simulink model "pv_wind_hybrid"  (R2024a)
settings: Solver=VariableStepAuto  StartTime=0.0  StopTime=1  RelTol=1e-3
libraries: spsSeriesRLCBranchLib x24, spsIGBTDiodeLib x12, spsDiodeLib x7, spsSawtoothGeneratorLib x6, spsGroundLib x5, spsThreePhaseVIMeasurementLib x5, spsCurrentMeasurementLib x4, spsVoltageMeasurementLib x3, spspowerguiLib x2, spsIGBTLib x1, spsPVArrayLib x1, eePwmGenerator x1
settings Model: Creator=91889  LastModifiedBy=91889
settings SolverCC: ZeroCrossAlgorithm=Adaptive

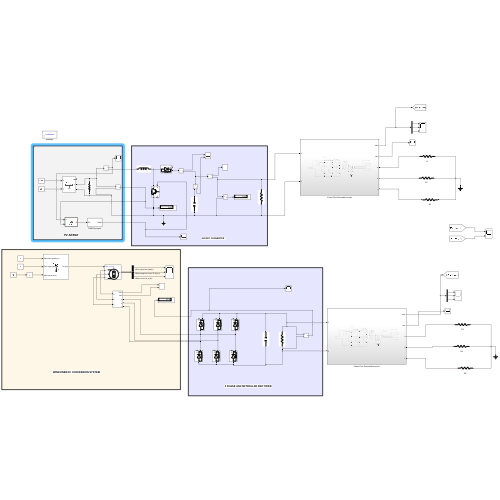
[thumbnail: Simulink's stored preview of the top-level diagram]
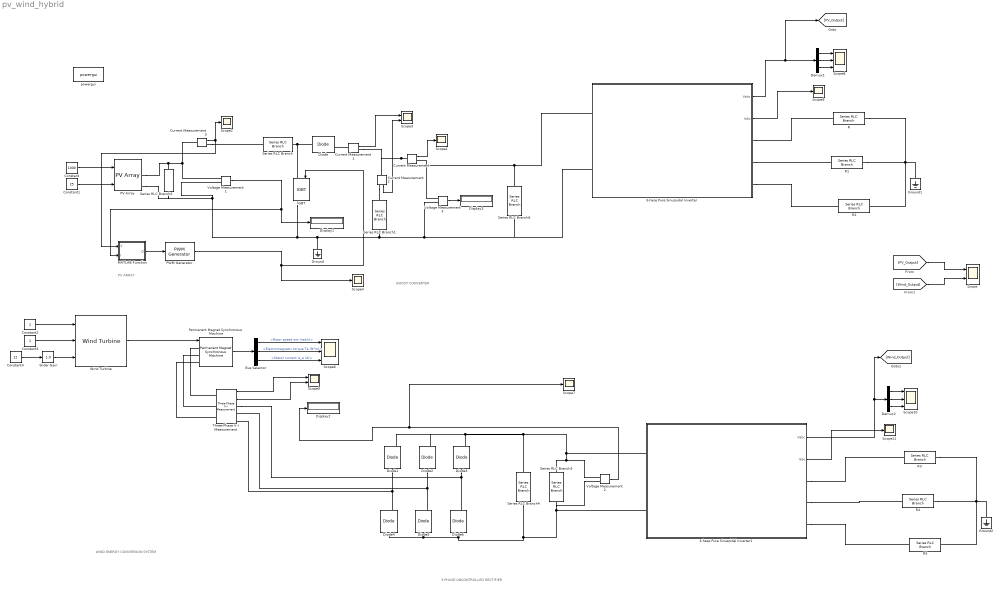
== system pv_wind_hybrid ==
  note: 3 PHASE UNCONTROLLED RECTIFIER
  note: WIND ENERGY CONVERSION SYSTEM
  note: BOOST CONVERTER
  note: PV ARRAY
  3-hase Pure Sinusoidal Inverter : Subsystem
  3-hase Pure Sinusoidal Inverter1 : Subsystem
  Bus Selector : BusSelector  OutputSignals=Rotor speed wm (rad/s),Electromagnetic torque Te (N*m),Stator current is_a (A)
  Constant : Constant  Value=1000
  Constant1 : Constant  Value=25
  Constant2 : Constant
  Constant3 : Constant
  Constant4 : Constant  Value=12
  Current Measurement{,1..3} (4 alike) : spsCurrentMeasurementLib/Current Measurement  PhasorSimulation=off  OutputType=Complex  PSBequivalent=0
  Demux1 : Demux  Outputs=3
  Demux2 : Demux  Outputs=3
  Diode{,1..6} (7 alike) : spsDiodeLib/Diode  Ron=0.001  Lon=0  Vf=0.8  IC=0  UseSnubber=0  Rs=500  Cs=250e-9  Measurements=on
  Display1 : Display
  Display2 : Display
  Display3 : Display
  Ground : spsGroundLib/Ground  LConnTagsString=a
  Ground1 : spsGroundLib/Ground  LConnTagsString=a
  Ground2 : spsGroundLib/Ground  LConnTagsString=a
  IGBT : spsIGBTLib/IGBT  Ron=0.001  Lon=0  Vf=1  Tf=1e-6  Tt=2e-6  IC=0  Rs=1e5  Cs=inf  Measurements=on
  MATLAB Function : MATLAB Function  TreatAsAtomicUnit=on
  PV Array : spsPVArrayLib/PV Array  Npar=1  Nser=1  PlotType=array @ 1000 W/m2 & specified temperatures  S_vec="[ 1000  500  100 ]"  Temp_C_vec="[ 45 25  ]"  ModuleName=User-defined  PlotWhenSelected=off  Pm=39.648  Ncell=36  Voc=21.6  Isc=2.55  Vm=16.8  Im=2.36  beta_Voc_pc=-0.36099  alpha_Isc_pc=0.102  beta_Voc=-0.077974  alpha_Isc=0.002601  IL=2.5568  I0=9.4856e-11  nI=0.97333  Rsh=355.4065  Rs=0.94376  RobustModel=off  RobustCellTemperature=313.3991  BAL=on  Tc=1e-6  Tfilter=5e-5
      link override Diode Rsh/Transfer Fcn: Numerator=10  Denominator=5e-1
  PWM Generator : eePwmGenerator/PWM Generator  CarrCount=Up  Tper=0.001  Tdelay=0  Ts=5e-5
  Permanent Magnet Synchronous Machine : spsPermanentMagnetSynchronousMachineLib/Permanent Magnet Synchronous Machine  NbPhases=3  FluxDistribution=Sinusoidal  RotorType=Round  MechanicalLoad=Torque Tm  PresetModel=No  ShowDetailedParameters=on  MeasurementBus=off  Resistance=0.0485  Inductance=8.5e-3  dqInductances=[8.5e-3,8.5e-3]  La=0.000395  MachineConstant=Flux linkage established by magnets (V.s)  Flux=0.1194  VoltageCst=86.6271  TorqueCst=0.7164  Flat=120  Mechanical=[0.0027 0.0004924 4 0]  PolePairs=4  InitialConditions=[0,0, 0,0]  InitialConditions5ph=[0 0 0 0 0 0]  RefAngle=90 degrees behind phase A axis (modified Park)  IterativeDiscreteModel=Trapezoidal non iterative  TsBlock=-1  TsPowergui=0
  R{,1..5} (6 alike) : spsSeriesRLCBranchLib/Series RLC Branch  LConnTagsString=__new0  RConnTagsString=__new0  BranchType=R  Resistance=10  Inductance=1e-3  SetiL0=off  InitialCurrent=0  Capacitance=1e-6  Setx0=off  InitialVoltage=0  Measurements=None
  Scope : Scope  NumInputPorts=2
  Scope{1..2,4,7,9,11} (6 alike) : Scope
  Scope10 : Scope  NumInputPorts=3
  Scope3 : Scope  NumInputPorts=2
  Scope5 : Scope  NumInputPorts=2
  Scope6 : Scope  NumInputPorts=3
  Scope8 : Scope  NumInputPorts=3
  Series RLC Branch : spsSeriesRLCBranchLib/Series RLC Branch  LConnTagsString=__new0  RConnTagsString=__new0  BranchType=L  Resistance=1  Inductance=32e-3  SetiL0=off  InitialCurrent=0  Capacitance=1e-6  Setx0=off  InitialVoltage=0  Measurements=None
  Series RLC Branch1 : spsSeriesRLCBranchLib/Series RLC Branch  LConnTagsString=__new0  RConnTagsString=__new0  BranchType=C  Resistance=1  Inductance=1e-3  SetiL0=off  InitialCurrent=0  Capacitance=1000e-6  Setx0=off  InitialVoltage=0  Measurements=None
  Series RLC Branch2 : spsSeriesRLCBranchLib/Series RLC Branch  LConnTagsString=__new0  RConnTagsString=__new0  BranchType=R  Resistance=200  Inductance=1e-3  SetiL0=off  InitialCurrent=0  Capacitance=1e-6  Setx0=off  InitialVoltage=0  Measurements=None
  Series RLC Branch3 : spsSeriesRLCBranchLib/Series RLC Branch  LConnTagsString=__new0  RConnTagsString=__new0  BranchType=R  Resistance=100  Inductance=1e-3  SetiL0=off  InitialCurrent=0  Capacitance=1e-6  Setx0=off  InitialVoltage=0  Measurements=None
  Series RLC Branch4 : spsSeriesRLCBranchLib/Series RLC Branch  LConnTagsString=__new0  RConnTagsString=__new0  BranchType=C  Resistance=1  Inductance=1e-3  SetiL0=off  InitialCurrent=0  Capacitance=1e-6  Setx0=off  InitialVoltage=0  Measurements=None
  Series RLC Branch6 : spsSeriesRLCBranchLib/Series RLC Branch  LConnTagsString=__new0  RConnTagsString=__new0  BranchType=R  Resistance=10  Inductance=1e-3  SetiL0=off  InitialCurrent=0  Capacitance=32e-6  Setx0=off  InitialVoltage=0  Measurements=None
  Slider Gain : simulink/Math Operations/Slider Gain  gain=1.0  low=0.5  high=1
  Three-Phase V-I Measurement : spsThreePhaseVIMeasurementLib/Three-Phase V-I Measurement  VoltageMeasurement=phase-to-phase  SetLabelV=off  LabelV=Vabc  Vpu=off  VpuLL=off  CurrentMeasurement=yes  SetLabelI=off  LabelI=Iabc  Ipu=off  Pbase=100e6  Vbase=500e3  OutputType=Complex  PhasorSimulation=off  PSBequivalent=0
  Voltage Measurement1 : spsVoltageMeasurementLib/Voltage Measurement  PhasorSimulation=off  OutputType=Complex  PSBequivalent=0
  Voltage Measurement2 : spsVoltageMeasurementLib/Voltage Measurement  PhasorSimulation=off  OutputType=Complex  PSBequivalent=0
  Voltage Measurement3 : spsVoltageMeasurementLib/Voltage Measurement  PhasorSimulation=off  OutputType=Complex  PSBequivalent=0
  Wind Turbine : spsWindTurbineLib/Wind Turbine  Pnom=1.5e6  Pelec_base=1.5e6/0.9  wind_base=12  P_wind_base=0.73  speed_nom=1.2  pitch_angle=0  c1_c6="[0.51763          116          0.4            5           21     0.006795]"  cp_nom=0.48  lambda_nom=8.1
  powergui : sps_lib/powergui  Priority=1  SimulationMode=Continuous  SampleTime=50e-6  frequency=60  Iterations=50  frequencyindice=0  Pbase=100e6  ErrMax=1e-4  UnitsV=kV  UnitsW=MW  buscounter=0  FunctionMessages=off  echomessages=off  EnableUseOfTLC=off  CurrentSourceSwitches=off  DisableSnubberDevices=off  DisableRonSwitches=off  DisableVfSwitches=off  DisplayEquations=off  AutomaticDiscreteSolvers=off  SolverType=Tustin/Backward Euler (TBE)  Interpol=off  ExternalGateDelay=off  methode=off  Ts=100  x0status=blocks  SPID=on  SwTol=0  HookPort=off  NonlinearTolerance=1e-4  nMaxIteration=100  ContinueOnMaxIteration=off  RestoreLinks=warning  ResistiveCurrentMeasurement=off  Frange=[0:2:500]  Ylog=off  Xlog=on  ShowGrid=off  save=off  variable=ZData  structure=0  ZoomFFT=off  StartTime=0.0  cycles=1  DisplayStyle=1  fundamental=60  FreqAxis=off  MaxFrequency=1000  frequencyindicesteady=1  RmsSteady=1  display=off
  wires:
  Current Measurement1/1 -> Scope3/1
  Current Measurement2/1 -> Scope3/2
  Current Measurement/1 -> Scope1/1
  Current Measurement3/1 -> Scope2/1, MATLAB Function/1(V)
  Constant/1 -> PV Array/1
  Constant1/1 -> PV Array/2
  Voltage Measurement1/1 -> MATLAB Function/2(I), Display1/1
  MATLAB Function/1(D) -> PWM Generator/1
  PWM Generator/1 -> Scope4/1, IGBT/1
  Bus Selector/2 -> Scope6/2  "<Electromagnetic torque Te (N*m)>"
  Bus Selector/3 -> Scope6/3  "<Stator current is_a (A)>"
  Constant4/1 -> Slider Gain/1
  Wind Turbine/1 -> Permanent Magnet Synchronous Machine/1
  Three-Phase V-I Measurement/2 -> Scope5/2
  Constant3/1 -> Wind Turbine/2
  Three-Phase V-I Measurement/1 -> Scope5/1
  Slider Gain/1 -> Wind Turbine/3
  Bus Selector/1 -> Scope6/1  "<Rotor speed wm (rad/s)>"
  Permanent Magnet Synchronous Machine/1 -> Bus Selector/1
  Constant2/1 -> Wind Turbine/1
  Voltage Measurement2/1 -> Display2/1, Scope7/1
  3-hase Pure Sinusoidal Inverter/2(Iabc) -> Scope9/1
  Demux1/3 -> Scope8/3
  Demux1/1 -> Scope8/1
  3-hase Pure Sinusoidal Inverter/1(Vabc) -> [PV_Output], Demux1/1
  Demux1/2 -> Scope8/2
  3-hase Pure Sinusoidal Inverter1/1(Vabc) -> [Wind_Output], Demux2/1
  Demux2/2 -> Scope10/2
  Demux2/3 -> Scope10/3
  Demux2/1 -> Scope10/1
  3-hase Pure Sinusoidal Inverter1/2(Iabc) -> Scope11/1
  Voltage Measurement3/1 -> Display3/1
  [PV_Output] -> Scope/1
  [Wind_Output] -> Scope/2
  connections:
  Series RLC Branch/RConn1 -- IGBT/LConn1 -- Diode/LConn1
  Current Measurement/LConn1 -- Current Measurement2/LConn1 -- Current Measurement1/RConn1
  Current Measurement3/RConn1 -- Series RLC Branch/LConn1
  Current Measurement1/LConn1 -- Diode/RConn1
  PV Array/RConn1 -- Series RLC Branch2/LConn1 -- Voltage Measurement1/LConn1 -- Current Measurement3/LConn1
  Current Measurement2/RConn1 -- Series RLC Branch1/LConn1
  Three-Phase V-I Measurement/LConn1 -- Permanent Magnet Synchronous Machine/LConn1
  Three-Phase V-I Measurement/LConn3 -- Permanent Magnet Synchronous Machine/LConn3
  Three-Phase V-I Measurement/LConn2 -- Permanent Magnet Synchronous Machine/LConn2
  Diode1/LConn1 -- Diode4/RConn1 -- Three-Phase V-I Measurement/RConn3
  Diode2/LConn1 -- Three-Phase V-I Measurement/RConn2 -- Diode5/RConn1
  Diode3/LConn1 -- Three-Phase V-I Measurement/RConn1 -- Diode6/RConn1
  Series RLC Branch3/LConn1 -- 3-hase Pure Sinusoidal Inverter1/LConn1 -- Series RLC Branch4/LConn1 -- Diode1/RConn1 -- Diode2/RConn1 -- Diode3/RConn1 -- Voltage Measurement2/LConn1
  IGBT/RConn1 -- Series RLC Branch2/RConn1 -- PV Array/RConn2 -- Voltage Measurement1/LConn2 -- Ground/LConn1 -- Series RLC Branch6/RConn1 -- 3-hase Pure Sinusoidal Inverter/LConn2 -- Voltage Measurement3/LConn2 -- Series RLC Branch1/RConn1
  R1/RConn1 -- R2/RConn1 -- Ground1/LConn1 -- R/RConn1
  3-hase Pure Sinusoidal Inverter/RConn1 -- R/LConn1
  3-hase Pure Sinusoidal Inverter/RConn2 -- R1/LConn1
  3-hase Pure Sinusoidal Inverter/RConn3 -- R2/LConn1
  R4/RConn1 -- R5/RConn1 -- Ground2/LConn1 -- R3/RConn1
  3-hase Pure Sinusoidal Inverter1/RConn3 -- R5/LConn1
  3-hase Pure Sinusoidal Inverter1/RConn2 -- R4/LConn1
  3-hase Pure Sinusoidal Inverter1/RConn1 -- R3/LConn1
  3-hase Pure Sinusoidal Inverter/LConn1 -- Series RLC Branch6/LConn1 -- Voltage Measurement3/LConn1 -- Current Measurement/RConn1
  3-hase Pure Sinusoidal Inverter1/LConn2 -- Series RLC Branch4/RConn1 -- Diode4/LConn1 -- Diode5/LConn1 -- Diode6/LConn1 -- Series RLC Branch3/RConn1 -- Voltage Measurement2/LConn2

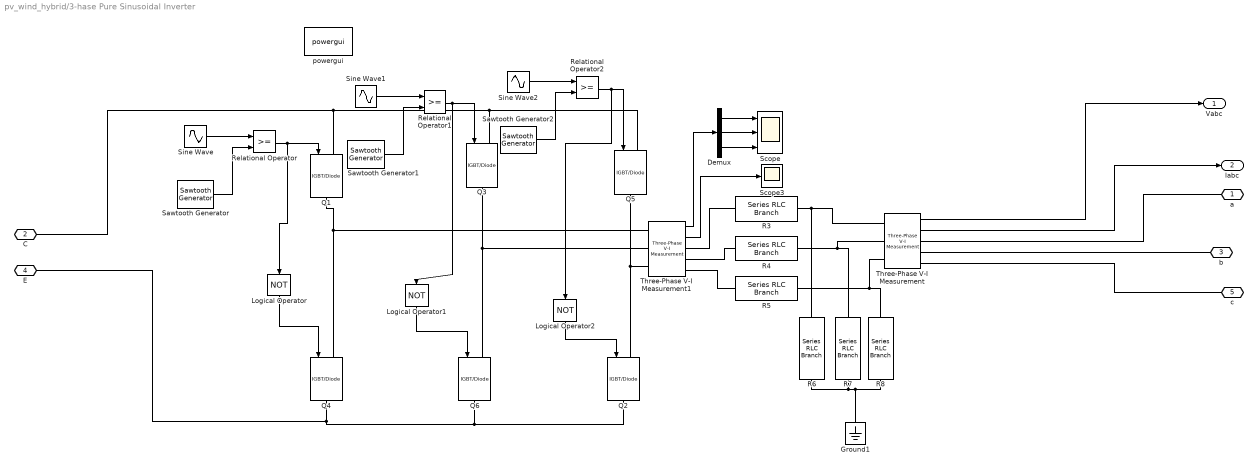
== system pv_wind_hybrid/3-hase Pure Sinusoidal Inverter ==
  Demux : Demux  Outputs=3
  Ground1 : spsGroundLib/Ground  LConnTagsString=a
  Logical Operator : Logic  Operator=NOT  AllPortsSameDT=off  OutDataTypeStr=boolean
  Logical Operator1 : Logic  Operator=NOT  AllPortsSameDT=off  OutDataTypeStr=boolean
  Logical Operator2 : Logic  Operator=NOT  AllPortsSameDT=off  OutDataTypeStr=boolean
  Q{1..6} (6 alike) : spsIGBTDiodeLib/IGBT//Diode  Ron=1e-3  Rs=1e5  Cs=inf  Measurements=off
  R3 : spsSeriesRLCBranchLib/Series RLC Branch  LConnTagsString=__new0  RConnTagsString=__new0  BranchType=L  Resistance=10  Inductance=80e-3  SetiL0=off  InitialCurrent=0  Capacitance=1e-6  Setx0=off  InitialVoltage=0  Measurements=None
  R4 : spsSeriesRLCBranchLib/Series RLC Branch  LConnTagsString=__new0  RConnTagsString=__new0  BranchType=L  Resistance=10  Inductance=80e-3  SetiL0=off  InitialCurrent=0  Capacitance=1e-6  Setx0=off  InitialVoltage=0  Measurements=None
  R5 : spsSeriesRLCBranchLib/Series RLC Branch  LConnTagsString=__new0  RConnTagsString=__new0  BranchType=L  Resistance=10  Inductance=80e-3  SetiL0=off  InitialCurrent=0  Capacitance=1e-6  Setx0=off  InitialVoltage=0  Measurements=None
  R6 : spsSeriesRLCBranchLib/Series RLC Branch  LConnTagsString=__new0  RConnTagsString=__new0  BranchType=C  Resistance=10  Inductance=80e-3  SetiL0=off  InitialCurrent=0  Capacitance=300e-6  Setx0=off  InitialVoltage=0  Measurements=None
  R7 : spsSeriesRLCBranchLib/Series RLC Branch  LConnTagsString=__new0  RConnTagsString=__new0  BranchType=C  Resistance=10  Inductance=80e-3  SetiL0=off  InitialCurrent=0  Capacitance=300e-6  Setx0=off  InitialVoltage=0  Measurements=None
  R8 : spsSeriesRLCBranchLib/Series RLC Branch  LConnTagsString=__new0  RConnTagsString=__new0  BranchType=C  Resistance=10  Inductance=80e-3  SetiL0=off  InitialCurrent=0  Capacitance=300e-6  Setx0=off  InitialVoltage=0  Measurements=None
  Relational Operator : RelationalOperator  OutDataTypeStr=boolean  InputSameDT=off
  Relational Operator1 : RelationalOperator  OutDataTypeStr=boolean  InputSameDT=off
  Relational Operator2 : RelationalOperator  OutDataTypeStr=boolean  InputSameDT=off
  Sawtooth Generator : spsSawtoothGeneratorLib/Sawtooth Generator  Freq=1000  Phase=180  Ts=0
  Sawtooth Generator1 : spsSawtoothGeneratorLib/Sawtooth Generator  Freq=1000  Phase=180  Ts=0
  Sawtooth Generator2 : spsSawtoothGeneratorLib/Sawtooth Generator  Freq=1000  Phase=180  Ts=0
  Scope : Scope  NumInputPorts=3
  Scope3 : Scope
  Sine Wave : Sin  Amplitude=0.9  Frequency=2*pi*50  SampleTime=0
  Sine Wave1 : Sin  Amplitude=0.9  Frequency=2*pi*50  Phase=120*(pi/180)  SampleTime=0
  Sine Wave2 : Sin  Amplitude=0.9  Frequency=2*pi*50  Phase=240*(pi/180)  SampleTime=0
  Three-Phase V-I Measurement : spsThreePhaseVIMeasurementLib/Three-Phase V-I Measurement  VoltageMeasurement=phase-to-phase  SetLabelV=off  LabelV=Vabc  Vpu=off  VpuLL=off  CurrentMeasurement=yes  SetLabelI=off  LabelI=Iabc  Ipu=off  Pbase=100e6  Vbase=500e3  OutputType=Complex  PhasorSimulation=off  PSBequivalent=0
  Three-Phase V-I Measurement1 : spsThreePhaseVIMeasurementLib/Three-Phase V-I Measurement  VoltageMeasurement=phase-to-phase  SetLabelV=off  LabelV=Vabc  Vpu=off  VpuLL=off  CurrentMeasurement=yes  SetLabelI=off  LabelI=Iabc  Ipu=off  Pbase=100e6  Vbase=500e3  OutputType=Complex  PhasorSimulation=off  PSBequivalent=0
  powergui : spspowerguiLib/powergui  Priority=1  SimulationMode=Continuous  SampleTime=50e-6  frequency=60  Iterations=50  frequencyindice=0  Pbase=100e6  ErrMax=1e-4  UnitsV=kV  UnitsW=MW  buscounter=0  FunctionMessages=off  echomessages=off  EnableUseOfTLC=off  CurrentSourceSwitches=off  DisableSnubberDevices=off  DisableRonSwitches=off  DisableVfSwitches=off  DisplayEquations=off  AutomaticDiscreteSolvers=off  SolverType=Tustin/Backward Euler (TBE)  Interpol=off  ExternalGateDelay=off  methode=off  Ts=100  x0status=blocks  SPID=off  SwTol=0  HookPort=off  NonlinearTolerance=1e-4  nMaxIteration=100  ContinueOnMaxIteration=off  RestoreLinks=warning  ResistiveCurrentMeasurement=off  Frange=[0:2:500]  Ylog=off  Xlog=on  ShowGrid=off  save=off  variable=ZData  structure=Vo  ZoomFFT=off  StartTime=0.0  cycles=1  DisplayStyle=1  fundamental=50  FreqAxis=on  MaxFrequency=1000  frequencyindicesteady=1  RmsSteady=1  display=off
  a : PMIOPort  Side=Right
  C : PMIOPort  Port=2  Side=Left
  b : PMIOPort  Port=3  Side=Right
  E : PMIOPort  Port=4  Side=Left
  c : PMIOPort  Port=5  Side=Right
  Vabc : Outport
  Iabc : Outport  Port=2
  wires:
  Relational Operator1/1 -> Q3/1, Logical Operator1/1
  Logical Operator/1 -> Q4/1
  Three-Phase V-I Measurement/1 -> Vabc/1
  Three-Phase V-I Measurement1/2 -> Scope3/1
  Logical Operator1/1 -> Q6/1
  Sawtooth Generator2/1 -> Relational Operator2/2
  Relational Operator2/1 -> Logical Operator2/1, Q5/1
  Logical Operator2/1 -> Q2/1
  Sawtooth Generator/1 -> Relational Operator/2
  Demux/1 -> Scope/1
  Three-Phase V-I Measurement1/1 -> Demux/1
  Relational Operator/1 -> Logical Operator/1, Q1/1
  Sawtooth Generator1/1 -> Relational Operator1/2
  Sine Wave/1 -> Relational Operator/1
  Three-Phase V-I Measurement/2 -> Iabc/1
  Sine Wave1/1 -> Relational Operator1/1
  Sine Wave2/1 -> Relational Operator2/1
  Demux/3 -> Scope/3
  Demux/2 -> Scope/2
  connections:
  R4/LConn1 -- Three-Phase V-I Measurement1/RConn2
  Q4/RConn1 -- Q6/RConn1 -- Q2/RConn1 -- E/RConn1
  Q5/LConn1 -- Q3/LConn1 -- Q1/LConn1 -- C/RConn1
  R6/LConn1 -- Three-Phase V-I Measurement/LConn1 -- R3/RConn1
  Three-Phase V-I Measurement1/LConn3 -- Q5/RConn1 -- Q2/LConn1
  Three-Phase V-I Measurement1/LConn2 -- Q3/RConn1 -- Q6/LConn1
  R7/LConn1 -- R4/RConn1 -- Three-Phase V-I Measurement/LConn2
  R5/LConn1 -- Three-Phase V-I Measurement1/RConn3
  Ground1/LConn1 -- R8/RConn1 -- R6/RConn1 -- R7/RConn1
  R8/LConn1 -- R5/RConn1 -- Three-Phase V-I Measurement/LConn3
  Three-Phase V-I Measurement/RConn3 -- c/RConn1
  Three-Phase V-I Measurement1/LConn1 -- Q1/RConn1 -- Q4/LConn1
  R3/LConn1 -- Three-Phase V-I Measurement1/RConn1
  Three-Phase V-I Measurement/RConn1 -- a/RConn1
  Three-Phase V-I Measurement/RConn2 -- b/RConn1

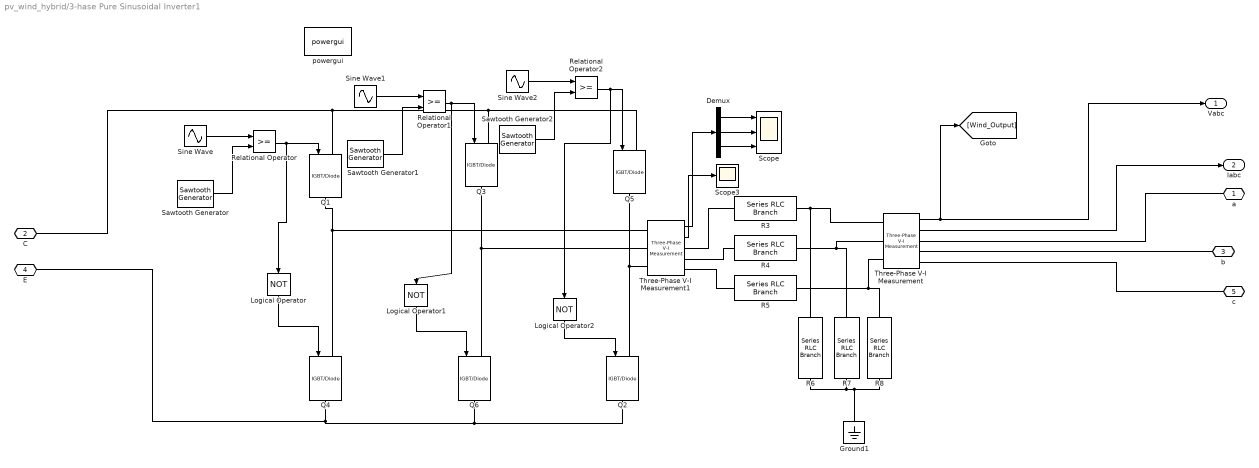
== system pv_wind_hybrid/3-hase Pure Sinusoidal Inverter1 ==
  Demux : Demux  Outputs=3
  Ground1 : spsGroundLib/Ground  LConnTagsString=a
  Logical Operator : Logic  Operator=NOT  AllPortsSameDT=off  OutDataTypeStr=boolean
  Logical Operator1 : Logic  Operator=NOT  AllPortsSameDT=off  OutDataTypeStr=boolean
  Logical Operator2 : Logic  Operator=NOT  AllPortsSameDT=off  OutDataTypeStr=boolean
  Q{1..6} (6 alike) : spsIGBTDiodeLib/IGBT//Diode  Ron=1e-3  Rs=1e5  Cs=inf  Measurements=off
  R3 : spsSeriesRLCBranchLib/Series RLC Branch  LConnTagsString=__new0  RConnTagsString=__new0  BranchType=L  Resistance=10  Inductance=80e-3  SetiL0=off  InitialCurrent=0  Capacitance=1e-6  Setx0=off  InitialVoltage=0  Measurements=None
  R4 : spsSeriesRLCBranchLib/Series RLC Branch  LConnTagsString=__new0  RConnTagsString=__new0  BranchType=L  Resistance=10  Inductance=80e-3  SetiL0=off  InitialCurrent=0  Capacitance=1e-6  Setx0=off  InitialVoltage=0  Measurements=None
  R5 : spsSeriesRLCBranchLib/Series RLC Branch  LConnTagsString=__new0  RConnTagsString=__new0  BranchType=L  Resistance=10  Inductance=80e-3  SetiL0=off  InitialCurrent=0  Capacitance=1e-6  Setx0=off  InitialVoltage=0  Measurements=None
  R6 : spsSeriesRLCBranchLib/Series RLC Branch  LConnTagsString=__new0  RConnTagsString=__new0  BranchType=C  Resistance=10  Inductance=80e-3  SetiL0=off  InitialCurrent=0  Capacitance=300e-6  Setx0=off  InitialVoltage=0  Measurements=None
  R7 : spsSeriesRLCBranchLib/Series RLC Branch  LConnTagsString=__new0  RConnTagsString=__new0  BranchType=C  Resistance=10  Inductance=80e-3  SetiL0=off  InitialCurrent=0  Capacitance=300e-6  Setx0=off  InitialVoltage=0  Measurements=None
  R8 : spsSeriesRLCBranchLib/Series RLC Branch  LConnTagsString=__new0  RConnTagsString=__new0  BranchType=C  Resistance=10  Inductance=80e-3  SetiL0=off  InitialCurrent=0  Capacitance=300e-6  Setx0=off  InitialVoltage=0  Measurements=None
  Relational Operator : RelationalOperator  OutDataTypeStr=boolean  InputSameDT=off
  Relational Operator1 : RelationalOperator  OutDataTypeStr=boolean  InputSameDT=off
  Relational Operator2 : RelationalOperator  OutDataTypeStr=boolean  InputSameDT=off
  Sawtooth Generator : spsSawtoothGeneratorLib/Sawtooth Generator  Freq=1000  Phase=180  Ts=0
  Sawtooth Generator1 : spsSawtoothGeneratorLib/Sawtooth Generator  Freq=1000  Phase=180  Ts=0
  Sawtooth Generator2 : spsSawtoothGeneratorLib/Sawtooth Generator  Freq=1000  Phase=180  Ts=0
  Scope : Scope  NumInputPorts=3
  Scope3 : Scope
  Sine Wave : Sin  Amplitude=0.9  Frequency=2*pi*50  SampleTime=0
  Sine Wave1 : Sin  Amplitude=0.9  Frequency=2*pi*50  Phase=120*(pi/180)  SampleTime=0
  Sine Wave2 : Sin  Amplitude=0.9  Frequency=2*pi*50  Phase=240*(pi/180)  SampleTime=0
  Three-Phase V-I Measurement : spsThreePhaseVIMeasurementLib/Three-Phase V-I Measurement  VoltageMeasurement=phase-to-phase  SetLabelV=off  LabelV=Vabc  Vpu=off  VpuLL=off  CurrentMeasurement=yes  SetLabelI=off  LabelI=Iabc  Ipu=off  Pbase=100e6  Vbase=500e3  OutputType=Complex  PhasorSimulation=off  PSBequivalent=0
  Three-Phase V-I Measurement1 : spsThreePhaseVIMeasurementLib/Three-Phase V-I Measurement  VoltageMeasurement=phase-to-phase  SetLabelV=off  LabelV=Vabc  Vpu=off  VpuLL=off  CurrentMeasurement=yes  SetLabelI=off  LabelI=Iabc  Ipu=off  Pbase=100e6  Vbase=500e3  OutputType=Complex  PhasorSimulation=off  PSBequivalent=0
  powergui : spspowerguiLib/powergui  Priority=1  SimulationMode=Continuous  SampleTime=50e-6  frequency=60  Iterations=50  frequencyindice=0  Pbase=100e6  ErrMax=1e-4  UnitsV=kV  UnitsW=MW  buscounter=0  FunctionMessages=off  echomessages=off  EnableUseOfTLC=off  CurrentSourceSwitches=off  DisableSnubberDevices=off  DisableRonSwitches=off  DisableVfSwitches=off  DisplayEquations=off  AutomaticDiscreteSolvers=off  SolverType=Tustin/Backward Euler (TBE)  Interpol=off  ExternalGateDelay=off  methode=off  Ts=100  x0status=blocks  SPID=off  SwTol=0  HookPort=off  NonlinearTolerance=1e-4  nMaxIteration=100  ContinueOnMaxIteration=off  RestoreLinks=warning  ResistiveCurrentMeasurement=off  Frange=[0:2:500]  Ylog=off  Xlog=on  ShowGrid=off  save=off  variable=ZData  structure=Vo  ZoomFFT=off  StartTime=0.0  cycles=1  DisplayStyle=1  fundamental=50  FreqAxis=on  MaxFrequency=1000  frequencyindicesteady=1  RmsSteady=1  display=off
  a : PMIOPort  Side=Right
  C : PMIOPort  Port=2  Side=Left
  b : PMIOPort  Port=3  Side=Right
  E : PMIOPort  Port=4  Side=Left
  c : PMIOPort  Port=5  Side=Right
  Vabc : Outport
  Iabc : Outport  Port=2
  wires:
  Relational Operator1/1 -> Q3/1, Logical Operator1/1
  Logical Operator/1 -> Q4/1
  Three-Phase V-I Measurement/1 -> [Wind_Output], Vabc/1
  Three-Phase V-I Measurement1/2 -> Scope3/1
  Logical Operator1/1 -> Q6/1
  Sawtooth Generator2/1 -> Relational Operator2/2
  Relational Operator2/1 -> Logical Operator2/1, Q5/1
  Logical Operator2/1 -> Q2/1
  Sawtooth Generator/1 -> Relational Operator/2
  Demux/1 -> Scope/1
  Three-Phase V-I Measurement1/1 -> Demux/1
  Relational Operator/1 -> Logical Operator/1, Q1/1
  Sawtooth Generator1/1 -> Relational Operator1/2
  Sine Wave/1 -> Relational Operator/1
  Three-Phase V-I Measurement/2 -> Iabc/1
  Sine Wave1/1 -> Relational Operator1/1
  Sine Wave2/1 -> Relational Operator2/1
  Demux/3 -> Scope/3
  Demux/2 -> Scope/2
  connections:
  R4/LConn1 -- Three-Phase V-I Measurement1/RConn2
  Q4/RConn1 -- Q6/RConn1 -- Q2/RConn1 -- E/RConn1
  Q5/LConn1 -- Q3/LConn1 -- Q1/LConn1 -- C/RConn1
  R6/LConn1 -- Three-Phase V-I Measurement/LConn1 -- R3/RConn1
  Three-Phase V-I Measurement1/LConn3 -- Q5/RConn1 -- Q2/LConn1
  Three-Phase V-I Measurement1/LConn2 -- Q3/RConn1 -- Q6/LConn1
  R7/LConn1 -- R4/RConn1 -- Three-Phase V-I Measurement/LConn2
  R5/LConn1 -- Three-Phase V-I Measurement1/RConn3
  Ground1/LConn1 -- R8/RConn1 -- R6/RConn1 -- R7/RConn1
  R8/LConn1 -- R5/RConn1 -- Three-Phase V-I Measurement/LConn3
  Three-Phase V-I Measurement/RConn3 -- c/RConn1
  Three-Phase V-I Measurement1/LConn1 -- Q1/RConn1 -- Q4/LConn1
  R3/LConn1 -- Three-Phase V-I Measurement1/RConn1
  Three-Phase V-I Measurement/RConn1 -- a/RConn1
  Three-Phase V-I Measurement/RConn2 -- b/RConn1

== matlab function pv_wind_hybrid/MATLAB Function ==
  settings: updateMethod=DISCRETE
  data: V input; D output; I input
function D = PnO(V, I)
% Persistent variables to store previous values
persistent V_prev I_prev P_prev D_prev direction

% Initialization
if isempty(V_prev)
    V_prev = 0; I_prev = 0; P_prev = 0; D_prev = 0.5; direction = 1;
end

% Current power
P = V * I;

% Compare current and previous power
if P > P_prev
    % Continue in same direction
    D = D_prev + 0.01 * direction;
else
    % Reverse direction
    direction = -direction;
    D = D_prev + 0.01 * direction;
end

% Clamp duty cycle between 0 and 1
D = max(min(D, 0.95), 0.05);

% Update persistent variables
V_prev = V;
I_prev = I;
P_prev = P;
D_prev = D;
end
